simulink model "modelling_lin"  (R2023b)
settings: Solver=VariableStepAuto  StartTime=0.0  StopTime=aero_p.simtime  RelTol=1e-3
undefined symbols (not defined in the file or in its folder): aero_lin_model, aero_p
settings Model: Creator=ben83  LastModifiedBy=ben83

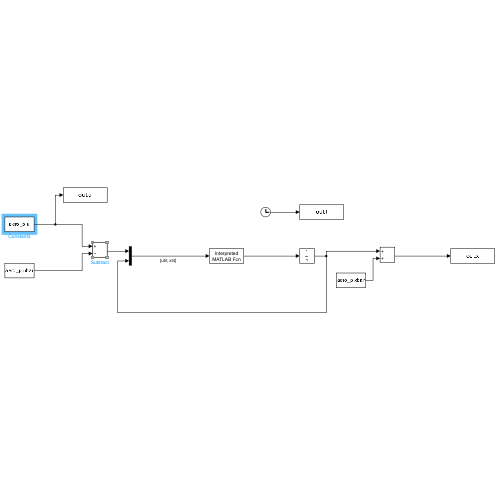
[thumbnail: Simulink's stored preview of the top-level diagram]
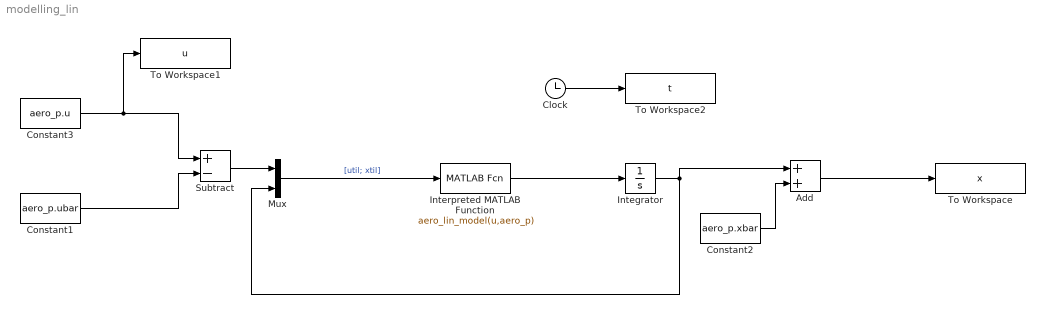
== system modelling_lin ==
  Add : Sum
  Clock : Clock
  Constant1 : Constant  Value=aero_p.ubar
  Constant2 : Constant  Value=aero_p.xbar
  Constant3 : Constant  Value=aero_p.u
  Integrator : Integrator  InitialCondition=aero_p.iclin
  Interpreted MATLAB Function : MATLABFcn  MATLABFcn=aero_lin_model(u,aero_p)
  Mux : Mux  Inputs=2
  Subtract : Sum  Inputs=+-
  To Workspace : ToWorkspace  VariableName=x  SampleTime=-1
  To Workspace1 : ToWorkspace  VariableName=u  SampleTime=-1
  To Workspace2 : ToWorkspace  VariableName=t  SampleTime=-1
  wires:
  Interpreted MATLAB Function/1 -> Integrator/1
  Mux/1 -> Interpreted MATLAB Function/1  "[util; xtil]"
  Clock/1 -> To Workspace2/1
  Integrator/1 -> Add/1, Mux/2
  Subtract/1 -> Mux/1
  Constant3/1 -> To Workspace1/1, Subtract/1
  Constant1/1 -> Subtract/2
  Add/1 -> To Workspace/1
  Constant2/1 -> Add/2
